simulink model "flightControlSystem"  (R2023a)
settings: Solver=ode3  StartTime=0  StopTime=TFinal  FixedStep=Ts  RelTol=1e-3  EnableMultiTasking=on
undefined symbols (not defined in the file): Centro_circulo, codertarget, Controller, DiscIntNeverNeededParam, Discrete, Estimator, g, gray, init, orient_ref, pos_ref, Sensors, Time, Ts, var_acc_angle_N, var_bias_gyr_N, var_gyro_p_N, Vehicle
libraries: simulink x38, slpidlib x4, simulink_extras x4, ctrlSharedLib x4, sharedtransform x3, visiontextngfix x3, visionstatistics x2, visiongeotforms x2, parrotlib x1
(part 3 of 3)

== system flightControlSystem/Control System/State Estimator/XY Position Estimator/EstimatorVelocity/xy velocity w//o angular velocity compensation ==
  note: Optical flow raw readings are converted to velocity in m/s based on the estimated altitude
  optical_flow : Inport
  z_estimate : Inport  Port=2
  " " : Product  Inputs=**
  Compare To Constant : simulink/Logic and Bit Operations/Compare To Constant  relop=<  const=200*4  OutDataTypeStr=boolean
  Counter Free-Running : simulink/Sources/Counter Free-Running  NumBits=32  tsamp=-1
  Gain : Gain  Gain=-1
  Select dxy : Selector  InputPortWidth=3  IndexOptions=Index vector (dialog)  Indices=[1 2]  OutputSizes=1
  Switch : Switch  Criteria=u2 > Threshold  SaturateOnIntegerOverflow=off  InputSameDT=off
  opticalFlowErrorCorrect : Gain  Gain=1.15
  optical_flow_dx_dy : Outport
  wires:
  Select dxy/1 -> optical_flow_dx_dy/1  "optical_flow_dx_dy"
  " "/1 -> opticalFlowErrorCorrect/1
  opticalFlowErrorCorrect/1 -> Switch/3
  Gain/1 -> " "/2
  Switch/1 -> Select dxy/1
  Counter Free-Running/1 -> Compare To Constant/1
  Compare To Constant/1 -> Switch/2
  optical_flow/1 -> " "/1, Switch/1
  z_estimate/1 -> Gain/1

== matlab function flightControlSystem/Image Processing System/Calibrate for Sim ==
  data: RGB input; maskedRGBImage output; BW output
function [maskedRGBImage, BW]= createMask(RGB)

%createMask  Threshold RGB image using auto-generated code from colorThresholder app.
%  [BW,MASKEDRGBIMAGE] = createMask(RGB) thresholds image RGB using
%  auto-generated code from the colorThresholder app. The colorspace and
%  range for each channel of the colorspace were set within the app. The
%  segmentation mask is returned in BW, and a composite of the mask and
%  original RGB images is returned in maskedRGBImage.

% Auto-generated by colorThresholder app on 27-Sep-2023
%------------------------------------------------------


% Convert RGB image to chosen color space
I = RGB;

% % Real Values
% channel1Min = 244.000;
% channel1Max = 255.000;
% channel2Min = 190.000;
% channel2Max = 255.000;
% channel3Min = 127.000;
% channel3Max = 255.000;


%Sim Values
channel1Min = 22.000;
channel1Max = 255.000;
channel2Min = 0.000;
channel2Max = 17.000;
channel3Min = 0.000;
channel3Max = 25.000;




% Create mask based on chosen histogram thresholds
sliderBW = (I(:,:,1) >= channel1Min ) & (I(:,:,1) <= channel1Max) & ...
    (I(:,:,2) >= channel2Min ) & (I(:,:,2) <= channel2Max) & ...
    (I(:,:,3) >= channel3Min ) & (I(:,:,3) <= channel3Max);
BW = sliderBW;

% Initialize output masked image based on input image.
maskedRGBImage = RGB;

% Set background pixels where BW is false to zero.
maskedRGBImage(repmat(~BW,[1 1 3])) = 0;

end

== matlab function flightControlSystem/Control System/Controller/Position Controller/Position error transformation (Earth to Body frame) ==
  data: yaw input; xy_err_earth input; xy_err_body output
function xy_err_body = fcn(yaw,xy_err_earth)

transformation = [cos(yaw), sin(yaw); -sin(yaw),  cos(yaw)];
xy_err_body = transformation * xy_err_earth;


end

== stateflow chart flightControlSystem/Control System/Path Planning/Chart ==
  state Moverse1
    entry:
    u = .4;
    v = .4;
    i= 0;
    during:
    xOut = 0;
    yOut = 0;
    zOut = -.9+i;
    i = i + .005;
  state Despegar
    entry:
    xOut = 0;
    yOut = 0;
    zOut = -.4;
    during:
    zOut = zEst -0.1;
  state Flotar
    entry:
    during:
    xOut = 0;
    yOut = 0;
    zOut = -.9;
    yaw_Out = .0;
  state Moverse
    entry:
    u = .7;
    v = .7;
    during:
    xOut = sind(c_theta)*u;
    yOut = cosd(c_theta)*v;
    zOut = -.9;
  (default) -> Despegar
  Moverse -> Moverse1 : [Circ_flag]
  Despegar -> Flotar : [zEst <= -.8]
  Flotar -> Moverse : after(3,sec)
  data: xOut output double; yOut output double; zOut output double; c_theta input; u local; v local; zEst input; yaw_Out output; Circ_flag input; i local

== matlab function flightControlSystem/Image Processing System/Mascara a rotar1 ==
  data: BW input; I output; C output; matCsup output; D output; giro output; threshold input
function [I,C,matCsup,D,giro] = fcn(BW, threshold)
giro = 0;
I = BW;
D = BW;
C = BW;
I(:,60:end) = 0;
C(:,[1:60, 120:end]) = 0; 
D(:,1:120) = 0;

matCsup = C;
matCsup(60:end,:) = 0;
Csup = sum(matCsup,"all")>threshold;
%Separar Izquierda en inferior y superior
matIsup = I;
matIsup(60:end,:) = 0;
Isup = sum(matIsup,"all")>threshold;

matIinf = I;
matIinf(1:70,:) = 0;
Iinf = sum(matIinf,"all")>threshold;
%Separar Derecha en inferior y superior
matDsup = D;
matDsup(60:end,:) = 0;
Dsup = sum(matDsup,"all")>threshold;

matDinf = D;
matDinf(1:70,:) = 0;
Dinf = sum(matDinf,"all")>threshold;


if Csup
    if Dsup
        if Dinf
            giro = .6;
        else
            giro = 1;
        end
    elseif Isup
        if Iinf
            giro = -.6;
        else
            giro = -1;
        end
    end
else
    giro = 0;
end

== matlab function flightControlSystem/Image Processing System/Mascara a rotar ==
  data: BW input; newBW output
function newBW = fcn(BW)
newBW = BW;
newBW(:,:) = 1;
max_pix = 120;
inicio = 45;
fin = 120-inicio;
% for c = 0:fin
%     b = c*max_pix/fin;
%     halfb = round(b/2);
%     newBW(inicio+c,80-halfb:80+halfb) = 0;
% end;

newBW(inicio:end,:) = 0;
newBW(1:inicio,1:30) = 0;
newBW(1:inicio,end-30:end) = 0;

== matlab function flightControlSystem/Image Processing System/Nuevo angulo ==
  data: p1 input; delta_x output; delta_y output; angle output; ccw_angle output
function [delta_x, delta_y, angle, ccw_angle] = fcn(p1)

center = [80,60];
delta_x = p1(1,1) - center(1);
delta_y = center(2) - p1(1,2);
if delta_x > 0
    if delta_y > 0
        angle = atand(delta_y/delta_x);
    else
        angle = 360 + atand(delta_y/delta_x);
    end;
else
    angle = atand(delta_y/delta_x)+180;
end;

if delta_x < 0
    if delta_y > 0
        ccw_angle = atand(delta_y/delta_x)+90;
    else
        ccw_angle = atand(delta_y/delta_x)+180;
    end;
else
    ccw_angle = atand(delta_y/delta_x)-90;
end;
